simulink library "UDPTouchpad"  (R2023b)
settings: Solver=VariableStepAuto  StartTime=0.0  StopTime=10.0  RelTol=1e-3
settings Model: Creator=Scythe  LastModifiedBy=Scythe

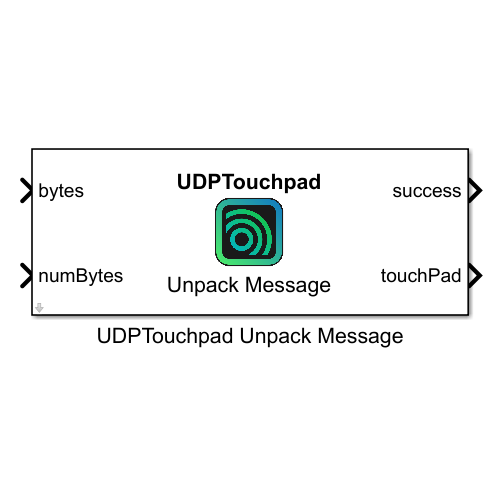
[thumbnail: Simulink's stored preview of the top-level diagram]
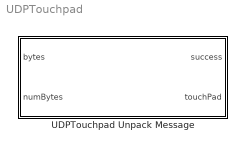
== system UDPTouchpad ==
  UDPTouchpad Unpack Message : Subsystem
      mask help: Unpack a binary message from the UDP touchpad app.
      mask DialogControl DescGroupVar Prompt: UDPTouchpad Unpack Message
      mask Display:
      | % Get dimension of block
      | pos = get_param(gcb, 'Position');
      | width = pos(3) - pos(1);
      | height = pos(4) - pos(2);
      | 
      | % Set image to center of block
      | imgSize = 32;
      | image('UDPTouchpad_Icon.svg', [0.5*(width-imgSize),0.5*(height-imgSize),imgSize,imgSize]);
      | 
      | % Block title
      | text(0.5*width,0.5*(height+imgSize)+2, '{\bfUDPTouchpad}','horizontalAlignment','center','verticalAlignment','bottom','texmode','on');
      | 
      | % Block name
      | text(0.5*width,0.5*(height-imgSize)-2,'Unpack Message', 'horizontalAlignment','center','verticalAlignment','top');

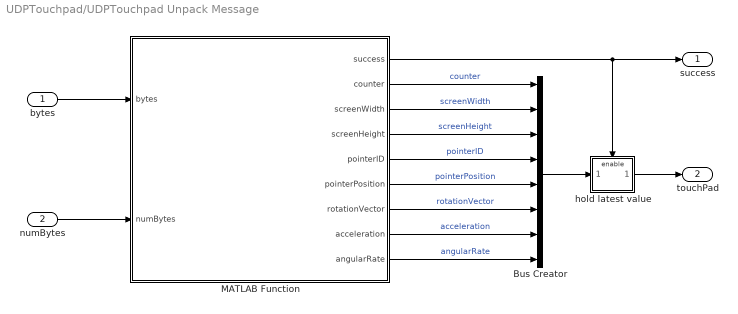
== system UDPTouchpad/UDPTouchpad Unpack Message ==
  bytes : Inport  OutDataTypeStr=uint8
  numBytes : Inport  Port=2  OutDataTypeStr=uint32  PortDimensions=1
  Bus Creator : BusCreator  Inputs=8
  MATLAB Function : MATLAB Function  TreatAsAtomicUnit=on
  hold latest value : Subsystem  TreatAsAtomicUnit=on
  success : Outport  OutDataTypeStr=boolean  PortDimensions=1
  touchPad : Outport  Port=2
  wires:
  bytes/1 -> MATLAB Function/1(bytes)
  numBytes/1 -> MATLAB Function/2(numBytes)
  MATLAB Function/5(pointerID) -> Bus Creator/4  "pointerID"
  Bus Creator/1 -> hold latest value/1(In1)
  MATLAB Function/2(counter) -> Bus Creator/1  "counter"
  MATLAB Function/9(angularRate) -> Bus Creator/8  "angularRate"
  MATLAB Function/6(pointerPosition) -> Bus Creator/5  "pointerPosition"
  MATLAB Function/8(acceleration) -> Bus Creator/7  "acceleration"
  MATLAB Function/1(success) -> success/1, hold latest value/Enable
  MATLAB Function/4(screenHeight) -> Bus Creator/3  "screenHeight"
  hold latest value/1(Out1) -> touchPad/1
  MATLAB Function/3(screenWidth) -> Bus Creator/2  "screenWidth"
  MATLAB Function/7(rotationVector) -> Bus Creator/6  "rotationVector"

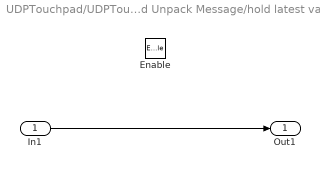
== system UDPTouchpad/UDPTouchpad Unpack Message/hold latest value ==
  In1 : Inport
  Enable : EnablePort
  Out1 : Outport
  wires:
  In1/1 -> Out1/1

== matlab function UDPTouchpad/UDPTouchpad Unpack Message/MATLAB Function ==
  data: bytes input uint8; success output boolean size=1; numBytes input uint32 size=1; counter output uint8 size=1; screenWidth output uint32 size=1; screenHeight output uint32 size=1; pointerID output uint8 size=10; pointerPosition output double size=[2,10]; rotationVector output double size=3; acceleration output double size=3; angularRate output double size=3
function [success,counter,screenWidth,screenHeight,pointerID,pointerPosition,rotationVector,acceleration,angularRate] = UnpackUDPTouchpad(bytes, numBytes)
    [success,result] = UDPTouchpad.UnpackMessage(bytes, numBytes);

    % set output values
    counter         = result.counter;
    screenWidth     = result.screenWidth;
    screenHeight    = result.screenHeight;
    pointerID       = result.pointerID;
    pointerPosition = result.pointerPosition;
    rotationVector  = result.rotationVector;
    acceleration    = result.acceleration;
    angularRate     = result.angularRate;
end
